simulink model "TestFlowAnyLength"  (R2013b)
settings: Solver=ode45  StartTime=0.0  StopTime=10.0  RelTol=1e-3
settings Model: Creator=qiji  LastModifiedBy=qiji

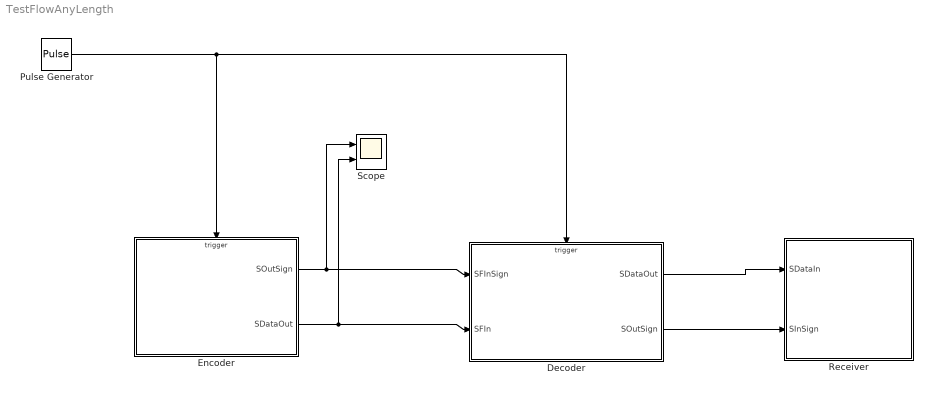
== system TestFlowAnyLength ==
  Decoder : Stateflow chart  TreatAsAtomicUnit=on
  Encoder : Stateflow chart  TreatAsAtomicUnit=on
  Pulse Generator : DiscretePulseGenerator  PulseType=Time based  Period=0.1  PulseWidth=50
  Receiver : Stateflow chart  TreatAsAtomicUnit=on
  Scope : Scope  NumInputPorts=2
      settings: YMin=-5~-5  YMax=5~5
  wires:
  Pulse Generator/1 -> Decoder/Trigger, Encoder/Trigger
  Encoder/2(SDataOut) -> Decoder/2(SFIn), Scope/2
  Encoder/1(SOutSign) -> Scope/1, Decoder/1(SFInSign)
  Decoder/1(SDataOut) -> Receiver/1(SDataIn)
  Decoder/2(SOutSign) -> Receiver/2(SInSign)

== stateflow chart TestFlowAnyLength/Encoder ==
  state judge
  state init [function]
    (default) -> (junction 19) : {
        | SFT[0][0] = 3;
        | SFT[0][1] = 10894;
        | SFT[0][2] = 12428;
        | SFT[0][3] = 19;
        | maxSize = 1;
        | SFCurrentIndex = 1;
        | SFIndex = 0;
        | count = 0;
        | SOutSign = false;
        | SOutSign = 0;
        | }
  state bitoperate [group]
  note: SOutSign = false后接收者才会开始读取
  state full
    full -> full [order 1] : CLK
        | {
        | SDataOut = bitoperate.getbit(input);
        | input = bitoperate.shiftbit(input, uint32(1));
        | count = count + 1;
        | }
  state empty
  judge -> empty [order 2] : {
      | SOutSign = false;
      | SFIndex++;
      | SFCurrentIndex = 1;
      | }
  full -> judge [order 1] : [count == 32]
      | {
      | SFCurrentIndex++;
      | }
  judge -> full [order 1] : [SFCurrentIndex<=SFT[SFIndex][0]]
      | {
      | count = 0;
      | input = ManchesterEncoding(SFT[SFIndex][SFCurrentIndex]);
      | }
  empty -> full : CLK[SFIndex < maxSize]
      | {
      | input = ManchesterEncoding(SFT[SFIndex][SFCurrentIndex]);
      | SOutSign = true;
      | SDataOut = 0;
      | count = 0;
      | }
  (default) -> empty : {
      | init();
      | }
  data: num function_input uint32; r function_output uint32; data function_input uint32; num function_input uint32; r function_output uint32; r function_output uint32; data function_input uint32; data function_input uint32; r function_output uint32; SFT local uint16 size=[2,5]; input local uint32; SFCurrentIndex local double; SFIndex local double; count local double; SOutSign output boolean; SDataOut output uint32; maxSize local double
  events: CLK input EITHER_EDGE_EVENT
  function r = getbit(num):
    | function r = getbit(num)
    | r = bitget(num, 32);
  function r = shiftbit(data, num):
    | function r = shiftbit(data, num)
    | r = bitshift(data, num);
    | %for i=1:cnt
    | %   r = bitset(r, i, 0);
    | %end
  function r = ManchesterDecoding(data):
    | function r = ManchesterDecoding(data)
    | r = uint32(0);
    | for i = (1:2:32)
    |     x0 = bitget(data, i);
    |     x1 = bitget(data, i+1);
    |     if x0==0 && x1==1
    |         r = bitset(r, (i+1)/2, 1);
    |     else
    |         r = bitset(r, (i+1)/2, 0);
    |     end
    | end
  function r = ManchesterEncoding(data):
    | function r = ManchesterEncoding(data)
    | r = data;
    | for i = 1:16
    |     x = bitget(data, i);
    |     if x == 0
    |         r = bitset(r, i*2-1, 1);
    |         r = bitset(r, i*2, 0);
    |     else
    |         r = bitset(r, i*2-1, 0);
    |         r = bitset(r, i*2, 1);
    |     end
    | end

== stateflow chart TestFlowAnyLength/Decoder ==
  state decodeSF
    decodeSF -> decodeSF [order 1] : CLK
        | {
        | ans = bitoperate.shiftbit(ans, 1) + SFIn;
        | count++;
        | }
  state bitoperate [group]
  state judge
    entry:
    ans = 0;
  state start
  decodeSF -> judge [order 1] : [count==32]
      | {
      | SDataOut = ManchesterDecoding(ans);
      | SOutSign = false;
      | count=0;
      | }
  start -> decodeSF : [SFInSign == true]
      | {
      | ans = 0;
      | count = 0;
      | SDataOut = 0;
      | ans = bitoperate.shiftbit(ans, 1) + SFIn;
      | SOutSign = true;
      | }
  judge -> decodeSF [order 1] : [SFInSign==true]
      | {
      | SOutSign = true;
      | }
  judge -> start [order 2]
  (default) -> start
  data: num function_input uint32; r function_output uint32; data function_input uint32; num function_input uint32; r function_output uint32; r function_output uint32; data function_input uint32; data function_input uint32; r function_output uint32; ans local uint32; count local double; SDataOut output uint32; SFInSign input boolean; SFIn input uint32; SOutSign output boolean
  events: CLK input EITHER_EDGE_EVENT
  function r = getbit(num):
    | function r = getbit(num)
    | r = bitget(num, 32);
  function r = shiftbit(data, num):
    | function r = shiftbit(data, num)
    | r = bitshift(data, num);
    | %for i=1:cnt
    | %   r = bitset(r, i, 0);
    | %end
  function r = ManchesterDecoding(data):
    | function r = ManchesterDecoding(data)
    | r = uint32(0);
    | for i = (1:2:32)
    |     x0 = bitget(data, i);
    |     x1 = bitget(data, i+1);
    |     if x0==0 && x1==1
    |         r = bitset(r, (i+1)/2, 1);
    |     else
    |         r = bitset(r, (i+1)/2, 0);
    |     end
    | end
  function r = ManchesterEncoding(data):
    | function r = ManchesterEncoding(data)
    | r = data;
    | for i = 1:16
    |     x = bitget(data, i);
    |     if x == 0
    |         r = bitset(r, i*2-1, 1);
    |         r = bitset(r, i*2, 0);
    |     else
    |         r = bitset(r, i*2-1, 0);
    |         r = bitset(r, i*2, 1);
    |     end
    | end

== stateflow chart TestFlowAnyLength/Receiver ==
  state bitoperate [group]
  state wait
  state trans
  state pushBack
  (default) -> wait : {
      | bufferIndex = 0;
      | }
  wait -> trans : [SInSign == true]
  pushBack -> wait
  trans -> pushBack : [SInSign== false]
      | {
      | buffer[bufferIndex] = SDataIn;
      | bufferIndex = bufferIndex + 1;
      | }
  data: num function_input uint32; r function_output uint32; data function_input uint32; num function_input uint32; r function_output uint32; r function_output uint32; data function_input uint32; data function_input uint32; r function_output uint32; SDataIn input uint32; buffer local uint16 size=10; bufferIndex local double; SInSign input boolean
  function r = getbit(num):
    | function r = getbit(num)
    | r = bitget(num, 32);
  function r = shiftbit(data, num):
    | function r = shiftbit(data, num)
    | r = bitshift(data, num);
    | %for i=1:cnt
    | %   r = bitset(r, i, 0);
    | %end
  function r = ManchesterDecoding(data):
    | function r = ManchesterDecoding(data)
    | r = uint32(0);
    | for i = (1:2:32)
    |     x0 = bitget(data, i);
    |     x1 = bitget(data, i+1);
    |     if x0==0 && x1==1
    |         r = bitset(r, (i+1)/2, 1);
    |     else
    |         r = bitset(r, (i+1)/2, 0);
    |     end
    | end
  function r = ManchesterEncoding(data):
    | function r = ManchesterEncoding(data)
    | r = data;
    | for i = 1:16
    |     x = bitget(data, i);
    |     if x == 0
    |         r = bitset(r, i*2-1, 1);
    |         r = bitset(r, i*2, 0);
    |     else
    |         r = bitset(r, i*2-1, 0);
    |         r = bitset(r, i*2, 1);
    |     end
    | end
